simulink model "simSystem_only_leader"  (R2022b)
settings: Solver=VariableStepAuto  StartTime=0.0  StopTime=60  RelTol=1e-3
values from neighbouring files (symbols this model uses):
  D_LIN = 1    [initFcn.m]
  D_QUAD = 1    [initFcn.m]
  M = M_RB + M_A    [initFcn.m]
undefined symbols (not defined in the file or in its folder): B, Continuous, I0, m, M_A, p, r_b_b, r_g_b, T, Time
libraries: simulink x2, aerolibguid x2, ctrlSharedLib x1
settings Model: Creator=User  LastModifiedBy=saigon
settings DebuggingCC: UnconnectedInputMsg=warning  UnconnectedOutputMsg=warning  UnconnectedLineMsg=warning
settings ModelReferenceCC: EnableRefExpFcnMdlSchedulingChecks=on
settings RTWCC: DLArmComputeVersion=19.05

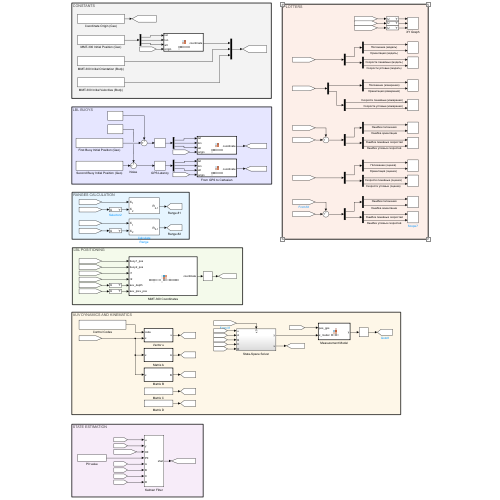
[thumbnail: Simulink's stored preview of the top-level diagram]
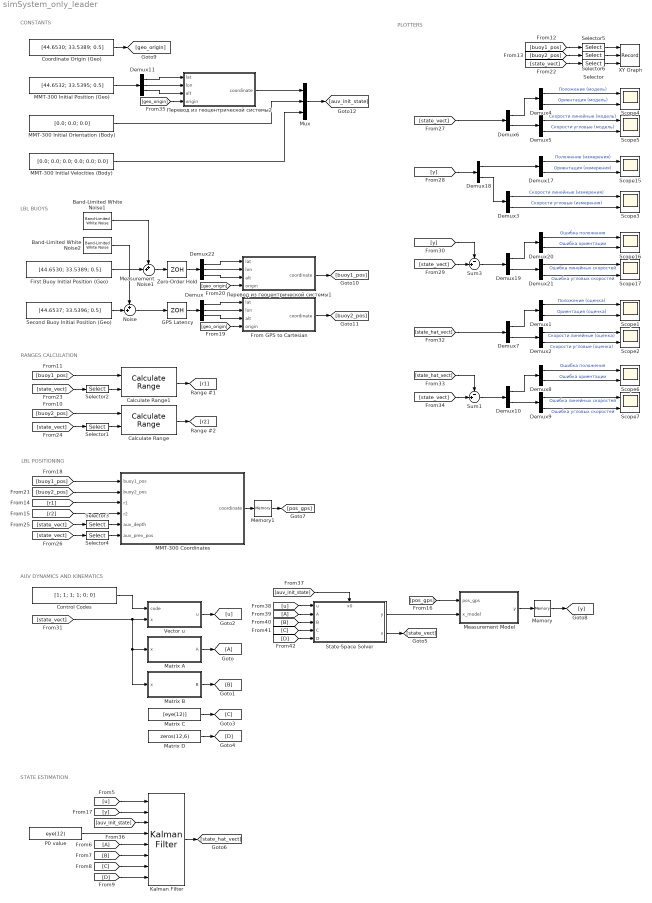
== system simSystem_only_leader ==
  note: PLOTTERS
  note: CONSTANTS
  note: STATE ESTIMATION
  note: AUV DYNAMICS AND KINEMATICS
  note: LBL POSITIONING
  note: RANGES CALCULATION
  note: LBL BUOYS
  Band-Limited White Noise1 : simulink/Sources/Band-Limited White Noise  Cov=[0.001; 0.001; 0] .* 0.00000001  Ts=0.1  seed=[23341]
  Band-Limited White Noise2 : simulink/Sources/Band-Limited White Noise  Cov=[0.0001; 0.0001; 0] .* 0.00000001  Ts=0.1  seed=[233341]
  Calculate Range : aerolibguid/Calculate Range
  Calculate Range1 : aerolibguid/Calculate Range
  Control Codes : Constant  Value=[1; 1; 1; 1; 0; 0]
  Coordinate Origin (Geo) : Constant  Value=[44.6530; 33.5389; 0.5]
  Demux : Demux  Outputs=3
  Demux{1..10,17..21} (15 alike) : Demux  Outputs=2
  Demux11 : Demux  Outputs=3
  Demux22 : Demux  Outputs=3
  First Buoy Initial Position (Geo) : Constant  Value=[44.6530; 33.5389; 0.5]
  From GPS to Cartesian : MATLAB Function  TreatAsAtomicUnit=on
  From39 : From
  From6 : From
  GPS Latency : ZeroOrderHold
  Goto : Goto
  Kalman Filter : ctrlSharedLib/Kalman Filter  TimeDomain=Continuous-Time  UseCurrentEstimator=on  ModelSource=Input port  ModelSourceVariable=ss(0.95,1,1,0,1)  A=0.95  B=1  C=1  D=0  NumberOfStates=12  NumberOfInputs=6  NumberOfOutputs=12  InitialEstimateSource=Input port  X0=0  P0=10  UseK=off  UseGH=off  NumberOfProcessNoiseInputs=1  G=1  TimeInvariantG=on  H=0  TimeInvariantH=on  Q=0  TimeInvariantQ=on  R=eye(12)  TimeInvariantR=on  N=0  TimeInvariantN=on  AddInputPort=on  AddEnablePort=off  OutputEstimatedY=off  OutputP=off  Ts=-1
  MMT-300 Coordinates : MATLAB Function  TreatAsAtomicUnit=on
  MMT-300 Initial Orientation (Body) : Constant  Value=[0.0; 0.0; 0.0]
  MMT-300 Initial Position (Geo) : Constant  Value=[44.6532; 33.5395; 0.5]
  MMT-300 Initial Velocities (Body) : Constant  Value=[0.0; 0.0; 0.0; 0.0; 0.0; 0.0]
  Matrix A : MATLAB Function  TreatAsAtomicUnit=on
  Matrix B : MATLAB Function  TreatAsAtomicUnit=on
  Matrix C : Constant  Value=[eye(12)]
  Matrix D : Constant  Value=zeros(12,6)
  Measurement Model : MATLAB Function  TreatAsAtomicUnit=on
  Measurement Noise1 : Sum  Inputs=++|
  Memory : Memory
  Memory1 : Memory
  Mux : Mux  Inputs=3
  Noise : Sum  Inputs=++|
  P0 value : Constant  Value=eye(12)
  Scope{1..7,15..17} (10 alike) : Scope  NumInputPorts=2
  Second Buoy Initial Position (Geo) : Constant  Value=[44.6537; 33.5396; 0.5]
  Selector : Selector  InputPortWidth=12  IndexOptions=Index vector (dialog)  Indices=[1 2]  OutputSizes=1
  Selector1 : Selector  InputPortWidth=12  IndexOptions=Index vector (dialog)  Indices=[1 2 3]  OutputSizes=1
  Selector2 : Selector  InputPortWidth=12  IndexOptions=Index vector (dialog)  Indices=[1 2 3]  OutputSizes=1
  Selector3 : Selector  InputPortWidth=12  IndexOptions=Index vector (dialog)  Indices=[3]  OutputSizes=1
  Selector4 : Selector  InputPortWidth=12  IndexOptions=Index vector (dialog)  Indices=[1 2]  OutputSizes=1
  Selector5 : Selector  InputPortWidth=3  IndexOptions=Index vector (dialog)  Indices=[1 2]  OutputSizes=1
  Selector6 : Selector  InputPortWidth=3  IndexOptions=Index vector (dialog)  Indices=[1 2]  OutputSizes=1
  State-Space Solver : Subsystem
      settings: PortSchema="{\"entries\":[{\"content\":{\"sides\":[{\"content\":{\"connectorIds\":[\"In1\",\"In2\",\"In3\",\"In4\",\"In5\"]},\"type\":\"ConnectorPlacement.EquallySpacedRectSide\",\"uuid\":\"3396e803-b255-47cb-93e0-45c7cfe2ef50\"},{\"content\":{\"connectorIds\":[\"Out1\",\"Out2\"],\"side\":\"RIGHT\"},\"type\":\"ConnectorPlacement.EquallySpacedRectSide\",\"uuid\":\"aa3f7afc-7592-49bf-8a0b-f10c1ca55260\"},{\"content\":{\"connectorIds\":[\"In6\"],\"side\":\"TOP\"},\"type\":\"ConnectorPlacement.EquallySpacedRectSide\",\"uuid\":\"2bd6e0b5-e2a0-49aa-8afc-b24b3510bd2d\"}]},\"type\":\"ConnectorPlacement.EquallySpacedConnector\",\"uuid\":\"56cebdc5-c080-4a47-a955-3b6265f64f70\"}],\"packageUris\":[\"http://schema.mathworks.com/mf0/Connector/R2020b\"],\"version\":\"1.0\"}"
  Sum1 : Sum  Inputs=-+|
  Sum3 : Sum  Inputs=-+|
  Vector u : MATLAB Function  TreatAsAtomicUnit=on
  XY Graph : Record  FileSettingsInternal="{\"entries\":[{\"content\":{\"excelSettings\":{\"content\":{},\"type\":\"Streamout.ExcelSettings\"}},\"type\":\"Streamout.FileSettingStorage\",\"uuid\":\"ec667d80-6cd4-4691-8339-9d7e799eb6ac\"}],\"packageUris\":[\"http://schema.mathworks.com/mf0/streamout_blocks/R2020a\"],\"version\":\"1.0\"}"  Layout=[1 1]  SignalsInternal="{\"entries\":[{\"content\":{\"signals\":[{\"content\":{\"blockPath\":[\"auv_simulink/XY Graph\"],\"channel\":[],\"dimensions\":[2],\"domain\":\"auv_simulink/XY Graph\",\"hasChildren\":true,\"lineColor\":\"#64d413\",\"plots\":[],\"port\":1,\"sid\":[\"\"],\"signalID\":4232,\"signalName\":\"Selector5\"},\"type\":\"RecordBlkView.Signal\",\"uuid\":\"80c9887f-3436-4141-83dd-de9e3ed14b6a\"},{\"content\":{\"blockPath\":[\"auv_simulink/XY Graph\"],\"channel\":[1],\"dimensions\":[2],\"domain\":\"auv_simulink/XY Graph\",\"lineColor\":\"#fe330a\",\"parentID\":4232,\"plots\":[1],\"port\":1,\"sid\":[\"\"],\"signalID\":4233,\"signalName\":\"Selector5\"},\"type\":\"RecordBlkView.Signal\",\"uuid\":\"9ed00e3e-211b-4476-b890-3916f39c209a\"},{\"content\":{\"blockPath\":[\"auv_simulink/XY Graph\"],\"channel\":[],\"dimensions\":[2],\"domain\":\"auv_simulink/XY Graph\",\"hasChildren\":true,\"lineColor\":\"#fe330a\",\"plots\":[],\"port\":2,\"sid\":[\"\"],\"signalID\":4237,\"signalName\":\"Selector6\"},\"type\":\"RecordBlkView.Signal\",\"uuid\":\"d9e2ab6a-b41b-456e-8fe5-e9b9dd68de05\"},{\"content\":{\"blockPath\":[\"auv_simulink/XY Graph\"],\"channel\":[1],\"dimensions\":[2],\"domain\":\"auv_simulink/XY Graph\",\"lineColor\":\"#0072bd\",\"parentID\":4237,\"plots\":[1],\"port\":2,\"sid\":[\"\"],\"signalID\":4238,\"signalName\":\"Selector6\"},\"type\":\"RecordBlkView.Signal\",\"uuid\":\"d0145706-67fc-4b54-95e3-2723d65c787c\"},{\"content\":{\"blockPath\":[\"auv_simulink/XY Graph\"],\"channel\":[],\"dimensions\":[2],\"domain\":\"auv_simulink/XY Graph\",\"hasChildren\":true,\"lineColor\":\"#0072bd\",\"plots\":[],\"port\":3,\"sid\":[\"\"],\"signalID\":4242,\"signalName\":\"Selector\"},\"type\":\"RecordBlkView.Signal\",\"uuid\":\"28d44f26-bb52-45d9-9db0-25437f38264c\"},{\"content\":{\"blockPath\":[\"auv_simulink/XY Graph\"],\"channel\":[1],\"dimensions\":[2],\"domain\":\"auv_simulink/XY Graph\",\"lineColor\":\"#7e2f8e\",\"parentID\":4242,\"plots\":[1],\"port\":3,\"sid\":[\"\"],\"signalID\":4243,\"signalName\":\"Selector\"},\"type\":\"RecordBlkView.Signal\",\"uuid\":\"d8409994-0bc7-482b-b849-1bca8afca5c8\"},{\"content\":{\"blockPath\":[\"auv_simulink/XY Graph\"],\"channel\":[2],\"dimensions\":[2],\"domain\":\"auv_simulink/XY Graph\",\"lineColor\":\"#edb120\",\"parentID\":4232,\"plots\":[1],\"port\":1,\"sid\":[\"\"],\"signalID\":4247,\"signalName\":\"Selector5\"},\"type\":\"RecordBlkView.Signal\",\"uuid\":\"2ce9df09-12f4-4b78-911a-19e65da7aa4f\"},{\"content\":{\"blockPath\":[\"auv_simulink/XY Graph\"],\"channel\":[2],\"dimensions\":[2],\"domain\":\"auv_simulink/XY Graph\",\"lineColor\":\"#7e2f8e\",\"parentID\":4237,\"plots\":[1],\"port\":2,\"sid\":[\"\"],\"signalID\":4248,\"signalName\":\"Selector6\"},\"type\":\"RecordBlkView.Signal\",\"uuid\":\"8d35fb3b-fd5d-43ae-992d-58763e4dc363\"},{\"content\":{\"blockPath\":[\"auv_simulink/XY Graph\"],\"channel\":[2],\"dimensions\":[2],\"domain\":\"auv_simulink/XY Graph\",\"lineColor\":\"#a2142f\",\"parentID\":4242,\"plots\":[1],\"port\":3,\"sid\":[\"\"],\"signalID\":4249,\"signalName\":\"Selector\"},\"type\":\"RecordBlkView.Signal\",\"uuid\":\"a2cc1dd4-291c-44a7-b47a-215f2a54a1f3\"}]},\"type\":\"RecordBlkView.InputSignals\",\"uuid\":\"a0ff2b65-1ff6-446e-bee3-eb09ad277175\"}],\"packageUris\":[\"http://schema.mathworks.com/mf0/streamout_blocks/R2020a\"],\"version\":\"1.0\"}"  VisualizationBindings="{\"xyplotplugin\":{\"info\":[{\"series\":[{\"bindingParametersList\":[{\"parameter\":\"X-Axis\",\"signalID\":4243,\"signalName\":\"Selector(1)\"},{\"parameter\":\"Y-Axis\",\"signalID\":4249,\"signalName\":\"Selector(2)\"}],\"seriesID\":21020},{\"bindingParametersList\":[{\"parameter\":\"X-Axis\",\"signalID\":4238,\"signalName\":\"Selector6(1)\"},{\"parameter\":\"Y-Axis\",\"signalID\":4248,\"signalName\":\"Selector6(2)\"}],\"seriesID\":577},{\"bindingParametersList\":[],\"seriesID\":39553},{\"bindingParametersList\":[],\"seriesID\":1647},{\"bindingParametersList\":[{\"parameter\":\"X-Axis\",\"signalID\":4233,\"signalName\":\"Selector5(1)\"},{\"parameter\":\"Y-Axis\",\"signalID\":4247,\"signalName\":\"Selector5(2)\"}],\"seriesID\":1088}],\"subplotID\":1}]}}"  CompatibilityTag=XY  st=-1
  Zero-Order Hold : ZeroOrderHold
  Перевод из геоцентрической системы1 : MATLAB Function  TreatAsAtomicUnit=on
  Перевод из геоцентрической системы2 : MATLAB Function  TreatAsAtomicUnit=on
  wires:
  P0 value/1 -> Kalman Filter/4
  Demux7/1 -> Demux1/1
  Demux7/2 -> Demux2/1
  Demux2/1 -> Scope2/1  "Скорости линейные (оценка)"
  Demux2/2 -> Scope2/2  "Скорости угловые (оценка)"
  Demux1/2 -> Scope1/2  "Ориентация (оценка)"
  Demux1/1 -> Scope1/1  "Положение (оценка)"
  Demux3/2 -> Scope3/2  "Скорости угловые (измерения)"
  Demux3/1 -> Scope3/1  "Скорости линейные (измерения)"
  State-Space Solver/1(y) -> Measurement Model/2(x_model)
  Demux4/1 -> Scope4/1  "Положение (модель)"
  Demux4/2 -> Scope4/2  "Ориентация (модель)"
  Demux5/2 -> Scope5/2  "Скорости угловые (модель)"
  Demux5/1 -> Scope5/1  "Скорости линейные (модель)"
  Demux6/2 -> Demux5/1
  Demux6/1 -> Demux4/1
  Demux10/1 -> Demux8/1
  Demux10/2 -> Demux9/1
  Sum1/1 -> Demux10/1
  Demux9/1 -> Scope7/1  "Ошибка линейных скоростей"
  Demux9/2 -> Scope7/2  "Ошибка угловых скоростей"
  Demux8/2 -> Scope6/2  "Ошибка ориентации"
  Demux8/1 -> Scope6/1  "Ошибка положения"
  Matrix A/1(A) -> Goto/1
  Matrix B/1(B) -> [B]
  Vector u/1(u) -> [u]
  Matrix C/1 -> [C]
  Matrix D/1 -> [D]
  [u] -> Kalman Filter/1
  From6/1 -> Kalman Filter/5
  [B] -> Kalman Filter/6
  [C] -> Kalman Filter/7
  [D] -> Kalman Filter/8
  [auv_init_state] -> Kalman Filter/3
  Selector/1 -> XY Graph/3
  Selector1/1 -> Calculate Range/2
  Calculate Range/1 -> [r2]
  Selector2/1 -> Calculate Range1/2
  Selector3/1 -> MMT-300 Coordinates/5(auv_depth)
  Selector4/1 -> MMT-300 Coordinates/6(auv_prev_pos)
  Calculate Range1/1 -> [r1]
  [buoy1_pos] -> Calculate Range1/1
  [buoy2_pos] -> Calculate Range/1
  [r1] -> MMT-300 Coordinates/3(r1)
  [r2] -> MMT-300 Coordinates/4(r2)
  MMT-300 Coordinates/1(coordinate) -> Memory1/1
  [pos_gps] -> Measurement Model/1(pos_gps)
  [y] -> Kalman Filter/2
  Measurement Model/1(y) -> Memory/1
  Demux17/2 -> Scope15/2  "Ориентация (измерения)"
  Demux17/1 -> Scope15/1  "Положение (измерения)"
  Demux18/2 -> Demux3/1
  Demux18/1 -> Demux17/1
  Memory/1 -> [y]
  Demux19/1 -> Demux20/1
  Demux19/2 -> Demux21/1
  Sum3/1 -> Demux19/1
  Demux21/1 -> Scope17/1  "Ошибка линейных скоростей"
  Demux21/2 -> Scope17/2  "Ошибка угловых скоростей"
  Demux20/2 -> Scope16/2  "Ошибка ориентации"
  Demux20/1 -> Scope16/1  "Ошибка положения"
  Memory1/1 -> [pos_gps]
  Control Codes/1 -> Vector u/1(code)
  Second Buoy Initial Position (Geo)/1 -> Noise/2
  Coordinate Origin (Geo)/1 -> [geo_origin]
  Noise/1 -> GPS Latency/1
  First Buoy Initial Position (Geo)/1 -> Measurement Noise1/2
  Measurement Noise1/1 -> Zero-Order Hold/1
  Band-Limited White Noise1/1 -> Measurement Noise1/1
  Band-Limited White Noise2/1 -> Noise/1
  GPS Latency/1 -> Demux/1
  Demux/1 -> From GPS to Cartesian/1(lat)
  Demux/2 -> From GPS to Cartesian/2(lon)
  Demux/3 -> From GPS to Cartesian/3(alt)
  Demux22/2 -> Перевод из геоцентрической системы1/2(lon)
  Demux22/1 -> Перевод из геоцентрической системы1/1(lat)
  Demux22/3 -> Перевод из геоцентрической системы1/3(alt)
  Zero-Order Hold/1 -> Demux22/1
  [geo_origin] -> From GPS to Cartesian/4(origin)
  [geo_origin] -> Перевод из геоцентрической системы1/4(origin)
  Перевод из геоцентрической системы1/1(coordinate) -> [buoy1_pos]
  From GPS to Cartesian/1(coordinate) -> [buoy2_pos]
  Selector5/1 -> XY Graph/1
  Selector6/1 -> XY Graph/2
  [buoy1_pos] -> Selector5/1
  [buoy2_pos] -> Selector6/1
  [buoy1_pos] -> MMT-300 Coordinates/1(buoy1_pos)
  [buoy2_pos] -> MMT-300 Coordinates/2(buoy2_pos)
  [state_vect] -> Selector/1
  [state_vect] -> Selector2/1
  [state_vect] -> Selector1/1
  [state_vect] -> Selector3/1
  [state_vect] -> Selector4/1
  State-Space Solver/2(x) -> [state_vect]
  [state_vect] -> Demux6/1
  [y] -> Demux18/1
  [state_vect] -> Sum3/2
  [y] -> Sum3/1
  [state_vect] -> Matrix B/1(x), Matrix A/1(x), Vector u/2(x)
  [state_hat_vect] -> Demux7/1
  [state_hat_vect] -> Sum1/1
  [state_vect] -> Sum1/2
  Kalman Filter/1 -> [state_hat_vect]
  [geo_origin] -> Перевод из геоцентрической системы2/4(origin)
  Demux11/2 -> Перевод из геоцентрической системы2/2(lon)
  Demux11/3 -> Перевод из геоцентрической системы2/3(alt)
  MMT-300 Initial Position (Geo)/1 -> Demux11/1
  Demux11/1 -> Перевод из геоцентрической системы2/1(lat)
  Mux/1 -> [auv_init_state]
  MMT-300 Initial Velocities (Body)/1 -> Mux/3
  MMT-300 Initial Orientation (Body)/1 -> Mux/2
  Перевод из геоцентрической системы2/1(coordinate) -> Mux/1
  [auv_init_state] -> State-Space Solver/6(x0)
  [D] -> State-Space Solver/5(D)
  [u] -> State-Space Solver/1(u)
  From39/1 -> State-Space Solver/2(A)
  [B] -> State-Space Solver/3(B)
  [C] -> State-Space Solver/4(C)

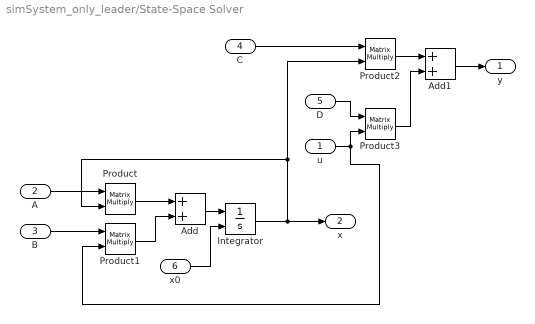
== system simSystem_only_leader/State-Space Solver ==
  u : Inport
  A : Inport  Port=2
  B : Inport  Port=3
  C : Inport  Port=4
  D : Inport  Port=5
  x0 : Inport  Port=6
  Add : Sum
  Add1 : Sum
  Integrator : Integrator  InitialConditionSource=external
  Product{,1..3} (4 alike) : Product  Multiplication=Matrix(*)
  y : Outport
  x : Outport  Port=2
  wires:
  x0/1 -> Integrator/2
  Integrator/1 -> Product/2, Product2/2, x/1
  A/1 -> Product/1
  B/1 -> Product1/1
  Product/1 -> Add/1
  Product1/1 -> Add/2
  Add/1 -> Integrator/1
  C/1 -> Product2/1
  Product2/1 -> Add1/1
  Product3/1 -> Add1/2
  D/1 -> Product3/1
  u/1 -> Product1/2, Product3/2
  Add1/1 -> y/1

== matlab function simSystem_only_leader/Перевод из геоцентрической системы2 ==
  data: lat input size=1 [-127..127]; lon input size=1; alt input size=1; origin input size=3; coordinate output size=3
function coordinate = geo2ned(lat, lon, alt, origin)
    coordinate = zeros(3,1);
    a = 6378137.0;
    b = 6356752.3142;
    B = deg2rad(lat);
    L = deg2rad(lon);
    H = alt;
    e2 = (a^2 - b^2) / a^2;
    NB = a / sqrt(1 - e2*sin(B)^2);
    x = (NB + H) * cos(B) * cos(L);
    y = (NB + H) * cos(B) * sin(L);
    z = ((b/a)^2 * NB + H) * sin(B);

    lat0 = origin(1);
    lon0 = origin(2);
    alt0 = origin(3);
    B = deg2rad(lat0);
    L = deg2rad(lon0);
    H = alt0;
    NB = a / sqrt(1 - e2*sin(B)^2);
    x0 = (NB + H) * cos(B) * cos(L);
    y0 = (NB + H) * cos(B) * sin(L);
    z0 = ((b/a)^2 * NB + H) * sin(B);

    xd = x - x0;
    yd = y - y0;
    zd = z - z0;
    
    coordinate(1) = -sin(L) * xd + cos(L) * yd;
    coordinate(2) = -cos(L) * sin(B) * xd - sin(B) * sin(L) * yd + cos(B) * zd;
    coordinate(3) = cos(B) * cos(L) * xd + cos(B) * sin(L) * yd + sin(B) * zd;

== matlab function simSystem_only_leader/Matrix A ==
  data: x input size=12; A output size=[12 12]; M parameter; I0 parameter; r_g_b parameter; m parameter; r_b_b parameter; M_A parameter; D_LIN parameter; D_QUAD parameter
function A = matrix_A(x, M, I0, r_g_b, m, r_b_b, M_A, D_LIN, D_QUAD)
n = 6;
eta = x(1:n); 
v = x(7:end);

%% ВСПОМОГАТЕЛЬНЫЕ ФУНКЦИИ
% преобразование в кососимметричную матрицу
S = @(x)([ 0 -x(3) x(2); x(3) 0 -x(1); -x(2) x(1) 0 ]); 

%% РАСЧЕТ ЯКОБИАНА
J_k_o = @(eta)[ 1  0           -sin(eta(5)); ...
                0  cos(eta(4))  cos(eta(5))*sin(eta(4)); ...
                0 -sin(eta(4))  cos(eta(5))*cos(eta(4)) ];
R_I_B = @(eta)[ cos(eta(6))*cos(eta(5))                                        sin(eta(6))*cos(eta(5))                                       -sin(eta(5)); ...
               -sin(eta(6))*cos(eta(4)) + cos(eta(6))*sin(eta(5))*sin(eta(4))  cos(eta(6))*cos(eta(4)) + sin(eta(6))*sin(eta(5))*sin(eta(4))  sin(eta(4))*cos(eta(5)); ...
                sin(eta(6))*sin(eta(4)) + cos(eta(6))*sin(eta(5))*cos(eta(4)) -cos(eta(6))*sin(eta(4)) + sin(eta(6))*sin(eta(5))*cos(eta(4))  cos(eta(4))*cos(eta(5)) ];
J = @(eta)[ R_I_B(eta) zeros(3); ...
            zeros(3)   J_k_o(eta) ];

%% РАСЧЕТ C(v)
% расчет C_RB(v)
%C_RB = @(v)([ zeros(3) -m*S(v(1:3)); -m*S(v(1:3)) -S(diag(I0).*v(4:end)) ]); 
C_RB = @(v)[ zeros(3)                           -m*S(v(1:3))-m*S(S(v(4:end))*r_g_b); ...
            -m*S(v(1:3))-m*S(S(v(4:end))*r_g_b)  m*S(S(v(1:3))*r_g_b)-S(I0*v(4:end)) ];
% расчет C_A(v)
diag_M_A = diag(M_A);
C_A = @(v)([ zeros(3) -S(diag_M_A(1:3).*v(1:3));
    -S(diag_M_A(1:3).*v(1:3)) -S(diag_M_A(4:end).*v(4:end))]);
% расчет C(v)
C = @(v)(C_RB(v) + C_A(v)); 
% M11 = M(1:3,1:3); M12 = M(1:3,4:6); M21 = M(4:6,1:3); M22 = M(4:6,4:6);
% C = @(v)[ zeros(3) -S(M11*v(1:3)+M12*v(4:6)); -S(M11*v(1:3)+M12*v(4:6)) -S(M21*v(1:3)+M22*v(4:6)) ];

%% РАСЧЕТ D(v)
%D = @(v)(abs(D_LIN) + abs(D_QUAD).*abs(v)); 
D = @(v)zeros(6,6);

A = [zeros(n), J(eta)^-1;
     zeros(n), -M^-1 * ( C(v) + D(v) )];

== matlab function simSystem_only_leader/Matrix B ==
  data: x input size=12; B output size=[12 6]; M parameter
function B = matrix_B(x, M)
n = 6;
B = [zeros(n); M^-1];

== matlab function simSystem_only_leader/Vector u ==
  data: code input [-127..127]; x input size=12; u output size=6; T parameter; p parameter; B parameter; m parameter; r_g_b parameter; r_b_b parameter
function u = vector_u(code,x, T, p, B, m, r_g_b, r_b_b)
n = 6;
eta = x(1:n); 

%% РАСЧЕТ g(n)
x_g = r_g_b(1); y_g = r_g_b(2); z_g = r_g_b(3);
x_b = r_b_b(1); y_b = r_b_b(2); z_b = r_b_b(3);
g = @(eta)[ (m*9.81-B)*sin(eta(5)); 
           -(m*9.81-B)*cos(eta(5))*sin(eta(4)); 
           -(m*9.81-B)*cos(eta(5))*cos(eta(4));
           -(y_g*m*9.81-y_b*B)*cos(eta(5))*cos(eta(4)) + ...
              (z_g*m*9.81-z_b*B)*cos(eta(5))*sin(eta(4));
            (z_g*m*9.81-z_b*B)*sin(eta(5)) + ...
              (x_g*m*9.81-x_b*B)*cos(eta(5))*cos(eta(4));
           -(x_g*m*9.81-x_b*B)*cos(eta(5))*sin(eta(4)) - ...
              (y_g*m*9.81-y_b*B)*sin(eta(5)) ]; 


F = @(code)polyval(p,code);

f1 = @(code)[ F(code)*cos(deg2rad(22)); 
              0; 
              F(code)*sin(deg2rad(22)) ];
f2 = @(code)[ F(code)*cos(deg2rad(22)); 
              F(code)*sin(deg2rad(22));
              0 ];
f3 = @(code)[ F(code)*cos(deg2rad(22)); 
              0; 
              -F(code)*sin(deg2rad(22)) ];
f4 = @(code)[ F(code)*cos(deg2rad(22));  
              -F(code)*sin(deg2rad(22));
              0 ];
f5 = @(code)[ 0; 
              F(code); 
              0 ];
f6 = @(code)[ 0; 
              0; 
              -F(code) ];

r1 = T(1,:)'; 
r2 = T(2,:)'; 
r3 = T(3,:)';
r4 = T(4,:)';
r5 = T(5,:)';
r6 = T(6,:)';
tau1 = @(code)[ f1(code); cross(r1, f1(code)) ];
tau2 = @(code)[ f2(code); cross(r2, f2(code)) ];
tau3 = @(code)[ f3(code); cross(r3, f3(code)) ];
tau4 = @(code)[ f4(code); cross(r4, f4(code)) ];
tau5 = @(code)[ f5(code); cross(r5, f5(code)) ];
tau6 = @(code)[ f6(code); cross(r6, f6(code)) ];

tau_c = @(code)[ tau1(code(1)), tau2(code(2)), tau3(code(3)), ...
                 tau4(code(4)), tau5(code(5)), tau6(code(6)) ];

thruster_mask = [1, 1, 1, 1, 1, 1]';

u = -g(eta) + tau_c(code) * thruster_mask;

== matlab function simSystem_only_leader/From GPS to Cartesian ==
  settings: updateMethod=DISCRETE
  data: lat input size=1 [-127..127]; lon input size=1; alt input size=1; origin input size=3; coordinate output size=3
function coordinate = geo2ned(lat, lon, alt, origin)
    coordinate = zeros(3,1);
    a = 6378137.0;
    b = 6356752.3142;
    B = deg2rad(lat);
    L = deg2rad(lon);
    H = alt;
    e2 = (a^2 - b^2) / a^2;
    NB = a / sqrt(1 - e2*sin(B)^2);
    x = (NB + H) * cos(B) * cos(L);
    y = (NB + H) * cos(B) * sin(L);
    z = ((b/a)^2 * NB + H) * sin(B);

    lat0 = origin(1);
    lon0 = origin(2);
    alt0 = origin(3);
    B = deg2rad(lat0);
    L = deg2rad(lon0);
    H = alt0;
    NB = a / sqrt(1 - e2*sin(B)^2);
    x0 = (NB + H) * cos(B) * cos(L);
    y0 = (NB + H) * cos(B) * sin(L);
    z0 = ((b/a)^2 * NB + H) * sin(B);

    xd = x - x0;
    yd = y - y0;
    zd = z - z0;
    coordinate(1) = -sin(L) * xd + cos(L) * yd;
    coordinate(2) = -cos(L) * sin(B) * xd - sin(B) * sin(L) * yd + cos(B) * zd;
    coordinate(3) = cos(B) * cos(L) * xd + cos(B) * sin(L) * yd + sin(B) * zd;

== matlab function simSystem_only_leader/Перевод из геоцентрической системы1 ==
  settings: updateMethod=DISCRETE
  data: lat input size=1 [-127..127]; lon input size=1; alt input size=1; origin input size=3; coordinate output size=3
function coordinate = geo2ned(lat, lon, alt, origin)
    coordinate = zeros(3,1);
    a = 6378137.0;
    b = 6356752.3142;
    B = deg2rad(lat);
    L = deg2rad(lon);
    H = alt;
    e2 = (a^2 - b^2) / a^2;
    NB = a / sqrt(1 - e2*sin(B)^2);
    x = (NB + H) * cos(B) * cos(L);
    y = (NB + H) * cos(B) * sin(L);
    z = ((b/a)^2 * NB + H) * sin(B);

    lat0 = origin(1);
    lon0 = origin(2);
    alt0 = origin(3);
    B = deg2rad(lat0);
    L = deg2rad(lon0);
    H = alt0;
    NB = a / sqrt(1 - e2*sin(B)^2);
    x0 = (NB + H) * cos(B) * cos(L);
    y0 = (NB + H) * cos(B) * sin(L);
    z0 = ((b/a)^2 * NB + H) * sin(B);

    xd = x - x0;
    yd = y - y0;
    zd = z - z0;
    coordinate(1) = -sin(L) * xd + cos(L) * yd;
    coordinate(2) = -cos(L) * sin(B) * xd - sin(B) * sin(L) * yd + cos(B) * zd;
    coordinate(3) = cos(B) * cos(L) * xd + cos(B) * sin(L) * yd + sin(B) * zd;

== matlab function simSystem_only_leader/MMT-300 Coordinates ==
  settings: updateMethod=DISCRETE
  data: buoy1_pos input size=3 [-127..127]; buoy2_pos input size=3; r1 input size=1; r2 input size=1; coordinate output size=2; auv_depth input size=1; auv_prev_pos input size=2
function coordinate = compute_coordinates(buoy1_pos, buoy2_pos, r1, r2, auv_depth, auv_prev_pos)
x_b1 = buoy1_pos(1); y_b1 = buoy1_pos(2); z_b1 = 0;
x_b2 = buoy2_pos(1); y_b2 = buoy2_pos(2); z_b2 = 0;

%% https://stackoverflow.com/questions/5238566/intersection-points-of-two-circles-in-matlab

A = [x_b1 y_b1]; %# center of the first circle
B = [x_b2 y_b2]; %# center of the second circle
a = sqrt(r2^2 - auv_depth^2); %# radius of the SECOND circle
b = sqrt(r1^2 - auv_depth^2); %# radius of the FIRST circle
c = norm(A-B); %# distance between circles

cosAlpha = (b^2+c^2-a^2)/(2*b*c);

u_AB = (B - A)/c; %# unit vector from first to second center
pu_AB = [u_AB(2), -u_AB(1)]; %# perpendicular vector to unit vector

%# use the cosine of alpha to calculate the length of the
%# vector along and perpendicular to AB that leads to the
%# intersection point
intersect_1 = A + u_AB * (b*cosAlpha) + pu_AB * (b*sqrt(1-cosAlpha^2));
intersect_2 = A + u_AB * (b*cosAlpha) - pu_AB * (b*sqrt(1-cosAlpha^2));

intersect_1 = intersect_1 + randn(1)/10;
intersect_2 = intersect_2 + randn(1)/10;

norm_est = [ norm([intersect_1(1) - auv_prev_pos(1), intersect_1(2) - auv_prev_pos(2)], 2); ...
             norm([intersect_2(1) - auv_prev_pos(1), intersect_2(2) - auv_prev_pos(2)], 2) ];

[~, idx] = min(norm_est);

if idx==1
    coordinate = intersect_1';
else
    coordinate = intersect_2';
end

== matlab function simSystem_only_leader/Measurement Model ==
  settings: updateMethod=DISCRETE
  data: pos_gps input size=2 [-127..127]; x_model input size=12; y output size=12
function y = MM(pos_gps, x_model)
pos_model = x_model(1:3); % imu + gps + pressure
ori_model = x_model(4:6); % imu
linvel_model = x_model(7:9); % imu + doppler
angvel_model = x_model(10:12); % imu

y = x_model;
y(1:2) = pos_gps;
y(3) = y(3) + randn(1) / 8;
y(4:6) = y(4:6) + randn(3,1) ./ 60;
y(7:9) = y(7:9) + randn(3,1) ./ 100;
y(9) = y(9) + randn(1) ./ 50;
y(10:12) = y(10:12) + randn(3,1) ./ 150;
